simulink model "DCmotor"  (Simulink 7.3)
settings: Solver=ode45  StartTime=0.0  StopTime=(N-1)*Ts  RelTol=1e-3
values from neighbouring files (symbols this model uses):
  Ts = 5E-3    (= 0.005)    [identification.m]
undefined symbols (not defined in the file or in its folder): Kb, Kt
libraries: dc_motor_lib x1
settings Model: Creator=Olov  LastModifiedBy=Olov

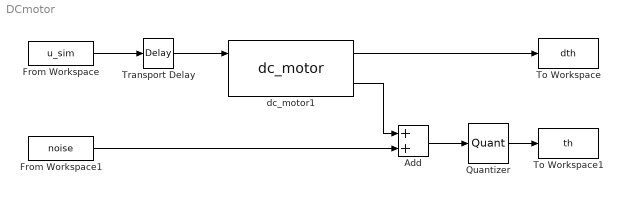
== system DCmotor ==
  Add : Sum  OutDataType=fixdt(1, 16)  OutScaling=2^-10
  From Workspace : FromWorkspace  VariableName=u_sim  SampleTime=Ts  Interpolate=off  OutputAfterFinalValue=Holding final value
  From Workspace1 : FromWorkspace  VariableName=noise  SampleTime=Ts  Interpolate=off  OutputAfterFinalValue=Holding final value
  Quantizer : Quantizer  QuantizationInterval=deg2rad(1)  LinearizeAsGain=off
  To Workspace : ToWorkspace  VariableName=dth  SampleTime=Ts  SaveFormat=Structure
  To Workspace1 : ToWorkspace  VariableName=th  SampleTime=Ts  SaveFormat=Structure
  Transport Delay : TransportDelay  DelayTime=Ts
  dc_motor1 : dc_motor_lib/dc_motor  SystemSampleTime=-1  Rm=Ra  Lm=0.000238  Kb=Kb  Kt=Kt  Jm=I  bm=Bm
  wires:
  From Workspace/1 -> Transport Delay/1
  dc_motor1/1 -> To Workspace/1
  Quantizer/1 -> To Workspace1/1
  dc_motor1/2 -> Add/1
  Add/1 -> Quantizer/1
  From Workspace1/1 -> Add/2
  Transport Delay/1 -> dc_motor1/1
